simulink model "H2_DRI_plant"  (R2023b)
settings: Solver=ode15s  StartTime=0.0  StopTime=3600*24*5
values from neighbouring files (symbols this model uses):
  a_b = 6*(1-eps_bed)/(r_p*2)    (= 200)    [H2_DRI_plant_loader.m]
  A_furnace = pi*r_furnace^2    (= 23.7582944428)    [H2_DRI_plant_loader.m]
  A_furnace_pel = A_furnace*(1-eps_bed)    (= 11.8791472214)    [H2_DRI_plant_loader.m]
  A_wall = (2*pi*r_furnace*dz)    (= 1.1674837564)    [H2_DRI_plant_loader.m]
  c_CH4init = interp1([1:1:length(c_CH4init)],c_CH4init, linspace(1,length(c_CH4init),n_furnace))    [H2_DRI_plant_loader.m]    (also in inital_conditions.m = out.CH4_conc.data(end,:); initcond_H2.mat = [9.94099064213e-45 -4.26076213273e-25 -4.27813906239e-25 -4.; initcond_H2_PEM.mat = [4.30667282687e-45 4.29087427587e-45 3.8700760922e-45 3.7994)
  c_Cinit = interp1([1:1:length(c_Cinit)],c_Cinit, linspace(1,length(c_Cinit),n_furnace))    [H2_DRI_plant_loader.m]    (also in inital_conditions.m = out.C_conc.data(end,:); initcond_H2.mat = [1.45956980986e-305 6.99081092012e-307 8.03725154841e-309 -3; initcond_H2_PEM.mat = [1.92191536232e-321 1.91203404941e-321 1.97132192691e-321 1.)
  c_CO2init = interp1([1:1:length(c_CO2init)],c_CO2init, linspace(1,length(c_CO2init),n_furnace))    [H2_DRI_plant_loader.m]    (also in inital_conditions.m = out.CO2_conc.data(end,:); initcond_H2.mat = [1.40671287015e-53 9.99429922421e-25 1.00349747704e-24 1.007; initcond_H2_PEM.mat = [4.30579616214e-45 4.28998535938e-45 3.86916279543e-45 3.798)
  c_COinit = interp1([1:1:length(c_COinit)],c_COinit, linspace(1,length(c_COinit),n_furnace))    [H2_DRI_plant_loader.m]    (also in inital_conditions.m = out.CO_conc.data(end,:); initcond_H2.mat = [8.62168160047e-54 2.62488347241e-25 2.63562031881e-25 2.646; initcond_H2_PEM.mat = [-1.41770643933e-43 -1.41248114323e-43 -1.27321677334e-43 -1)
  c_Fe2O3init = interp1([1:1:length(c_Fe2O3init)],c_Fe2O3init, linspace(1,length(c_Fe2O3init),n_furnace))    [H2_DRI_plant_loader.m]    (also in inital_conditions.m = out.Fe2O3_conc.data(end,:); initcond_H2.mat = [-0.0576294325141 -0.0562977053664 -0.0549879883395 -0.05369; initcond_H2_PEM.mat = [-0.0421766495112 -0.0410731169681 -0.0399918101679 -0.03893)
  c_Fe3O4init = interp1([1:1:length(c_Fe3O4init)],c_Fe3O4init, linspace(1,length(c_Fe3O4init),n_furnace))    [H2_DRI_plant_loader.m]    (also in inital_conditions.m = out.Fe3O4_conc.data(end,:); initcond_H2.mat = [0.0460784397936 0.0452182842983 0.0443654100081 0.043519007; initcond_H2_PEM.mat = [0.0345314201173 0.0338401633931 0.0331554273597 0.032476466)
  c_Feinit = interp1([1:1:length(c_Feinit)],c_Feinit, linspace(1,length(c_Feinit),n_furnace))    [H2_DRI_plant_loader.m]    (also in inital_conditions.m = out.Fe_conc.data(end,:); initcond_H2.mat = [2291.15615825 2257.57098555 2219.35021937 2176.85237423 213; initcond_H2_PEM.mat = [2291.15370188 2257.40533074 2219.07663621 2176.56351656 213)
  c_FeOinit = interp1([1:1:length(c_FeOinit)],c_FeOinit, linspace(1,length(c_FeOinit),n_furnace))    [H2_DRI_plant_loader.m]    (also in inital_conditions.m = out.FeO_conc.data(end,:); initcond_H2.mat = [120.587032003 163.793602795 212.96382844 267.636483226 327.; initcond_H2_PEM.mat = [120.587036941 164.003608886 213.312732219 268.005087273 327)
  c_H2init = interp1([1:1:length(c_H2init)],c_H2init, linspace(1,length(c_H2init),n_furnace))    [H2_DRI_plant_loader.m]    (also in inital_conditions.m = out.H2_conc.data(end,:); initcond_H2.mat = [22.889073739 22.8842667021 22.8746324515 22.8599710419 22.8; initcond_H2_PEM.mat = [17.1469199078 17.1645959742 17.1787956185 17.1891948084 17.)
  c_H2Oinit = interp1([1:1:length(c_H2Oinit)],c_H2Oinit, linspace(1,length(c_H2Oinit),n_furnace))    [H2_DRI_plant_loader.m]    (also in inital_conditions.m = out.H2O_conc.data(end,:); initcond_H2.mat = [2.19324064628 2.2939246227 2.40633645516 2.52967076126 2.66; initcond_H2_PEM.mat = [0.652099757837 0.728496202531 0.813916572535 0.907739128718)
  c_N2init = interp1([1:1:length(c_N2init)],c_N2init, linspace(1,length(c_N2init),n_furnace))    [H2_DRI_plant_loader.m]    (also in inital_conditions.m = out.N2_conc.data(end,:); initcond_H2.mat = [0.439764167248 0.441445162144 0.443247144888 0.445152489232; initcond_H2_PEM.mat = [0.271051060899 0.272483637209 0.274000693264 0.275587826454)
  CCeaf = CC_eaf*TPDls*365    (= 195258297.6)    [H2_DRI_plant_loader.m]
  CCelect = CC_elect*MWelect*1000    (= 420000000)    [H2_DRI_plant_loader.m]
  CCsf = 49080*(TPDls*DRIsteel_conv/24*1000)^(0.6538)    (= 108365944.556)    [H2_DRI_plant_loader.m]
  CO2_diff_prop = [MM_CO2, 26.9]    [H2_DRI_plant_loader.m]
  CO_diff_prop = [MM_CO, 18.9]    [H2_DRI_plant_loader.m]
  dz = (h_furnace/(n_furnace-1))    (= 0.0675675675676)    [H2_DRI_plant_loader.m]
  eps_bed = 0.5    [H2_DRI_plant_loader.m]
  H2_diff_prop = [MM_H2, 2.31*2]    [H2_DRI_plant_loader.m]
  H2O_diff_prop = [MM_H2O, 13.1]    [H2_DRI_plant_loader.m]
  H2only = true    [H2_DRI_plant_loader.m]
  I_metal = P_metal/tau_metal    (= -0.00212856534696)    [H2_DRI_plant_loader.m]
  I_temp = P_metal/tau_temp    (= -0.00681140911026)    [H2_DRI_plant_loader.m]
  Kd = 5.29e-4    (= 0.000529)    [H2_DRI_plant_loader.m]
  Kmetal = -0.0435    [H2_DRI_plant_loader.m]
  MM_C = 12.011/1000    (= 0.012011)    [H2_DRI_plant_loader.m]
  MM_CH4 = 16.04    [H2_DRI_plant_loader.m]
  MM_CO = 28.01    [H2_DRI_plant_loader.m]
  MM_CO2 = 44.01    [H2_DRI_plant_loader.m]
  MM_Fe = 55.845/1000    (= 0.055845)    [H2_DRI_plant_loader.m]    (also in iron_props.m)
  MM_Fe2O3 = 159.69/1000    (= 0.15969)    [H2_DRI_plant_loader.m]    (also in iron_props.m)
  MM_Fe3O4 = 231.53/1000    (= 0.23153)    [H2_DRI_plant_loader.m]    (also in iron_props.m = 0.25153)
  MM_FeO = 71.844/1000    (= 0.071844)    [H2_DRI_plant_loader.m]    (also in iron_props.m)
  MM_H2 = 2.016    [H2_DRI_plant_loader.m]
  MM_H2O = 18.015    [H2_DRI_plant_loader.m]
  MM_N2 = 28.013    [H2_DRI_plant_loader.m]
  n_furnace = 75    [H2_DRI_plant_loader.m]
  ndotin = 2078.874    [H2_DRI_plant_loader.m]
  nr1init = interp1([1:1:length(nr1init)],nr1init, linspace(1,length(nr1init),n_furnace))    [H2_DRI_plant_loader.m]    (also in inital_conditions.m = out.nr1.data(end,:); initcond_H2.mat = [17138.9259823 17138.9192887 17138.9127057 17138.9062259 171; initcond_H2_PEM.mat = [17138.8483125 17138.8427658 17138.8373309 17138.8319998 171)
  nr2init = interp1([1:1:length(nr2init)],nr2init, linspace(1,length(nr2init),n_furnace))    [H2_DRI_plant_loader.m]    (also in inital_conditions.m = out.nr2.data(end,:); initcond_H2.mat = [11425.7909148 11425.7894343 11425.7880023 11425.7866166 114; initcond_H2_PEM.mat = [11425.7791649 11425.7778635 11425.776614 11425.7754137 1142)
  nr3init = interp1([1:1:length(nr3init)],nr3init, linspace(1,length(nr3init),n_furnace))    [H2_DRI_plant_loader.m]    (also in inital_conditions.m = out.nr3.data(end,:); initcond_H2.mat = [32930.1678524 32447.4572478 31898.1205118 31287.3104766 306; initcond_H2_PEM.mat = [32930.1325476 32445.0763361 31894.188375 31283.1588034 3061)
  P_gin = 101325*1.8    (= 182385)    [H2_DRI_plant_loader.m]
  P_metal = tau_metal/(Kmetal*tau_metal_desired)    (= -24.5210727969)    [H2_DRI_plant_loader.m]
  P_temp = tau_temp/(Kmetal*tau_temp_desired)    (= -45.9770114943)    [H2_DRI_plant_loader.m]
  R = 8.314    [Bou.m]    (also in H2_DRI_plant_loader.m; MD.m; SMR.m; USCM_CO.m)
  r_furnace = 2.75    [H2_DRI_plant_loader.m]
  r_p = 15e-3/2    (= 0.0075)    [H2_DRI_plant_loader.m]
  rho_p = 3528    [H2_DRI_plant_loader.m]
  Solids_In_Flow = 44.1    [H2_DRI_plant_loader.m]
  T_gin = 947 + 273    (= 1220)    [H2_DRI_plant_loader.m]
  T_ginit = interp1([1:1:length(T_ginit)],T_ginit, linspace(1,length(T_ginit),n_furnace))    [H2_DRI_plant_loader.m]    (also in inital_conditions.m = out.T_g.data(end,2:end); initcond_H2.mat = [1193.47241077 1188.60147936 1183.4413554 1178.04610025 1172; initcond_H2_PEM.mat = [1213.62674902 1206.86882145 1199.80656651 1192.51337179 118)
  T_sin = -10 + 273    (= 263)    [H2_DRI_plant_loader.m]
  T_sinit = interp1([1:1:length(T_sinit)],T_sinit, linspace(1,length(T_sinit),n_furnace))    [H2_DRI_plant_loader.m]    (also in inital_conditions.m = out.T_s.data(end,1:end-1); initcond_H2.mat = [1188.32225462 1183.11411515 1177.66723955 1172.0331792 1166; initcond_H2_PEM.mat = [1207.76768382 1200.67884676 1193.34151616 1185.82650883 117)
  tau = 1    [H2_DRI_plant_loader.m]
  tau_d = 3600*2    (= 7200)    [H2_DRI_plant_loader.m]
  tau_metal = 3.2*3600    (= 11520)    [H2_DRI_plant_loader.m]
  V_g = (4/3)*pi*r_p^3*n_pellets_dz*(eps_bed/(1-eps_bed))    (= 0.802645082526)    [H2_DRI_plant_loader.m]
  V_p = 4/3*pi*r_p^3    (= 1.76714586764e-06)    [H2_DRI_plant_loader.m]
  V_s = (4/3)*pi*r_p^3*n_pellets_dz    (= 0.802645082526)    [H2_DRI_plant_loader.m]
  w_Cin = 0    [H2_DRI_plant_loader.m]
  w_Fe2O3in = 0.9665    [H2_DRI_plant_loader.m]
  w_Fe3O4in = 0    [H2_DRI_plant_loader.m]
  w_Fein = 0    [H2_DRI_plant_loader.m]
  w_FeOin = 0    [H2_DRI_plant_loader.m]
  w_Ganin = 0.0335    [H2_DRI_plant_loader.m]
  x_CH4in = 0.105824828    [H2_DRI_plant_loader.m]
  x_CO2in = 0.024    [H2_DRI_plant_loader.m]
  x_COin = 0.320711862    [H2_DRI_plant_loader.m]
  x_H2in = 0.489526511    [H2_DRI_plant_loader.m]
  x_H2Oin = 0.042557156    [H2_DRI_plant_loader.m]
  x_N2in = 0.017379642    [H2_DRI_plant_loader.m]
libraries: slpidlib x3, simulink x1
(part 2 of 3)

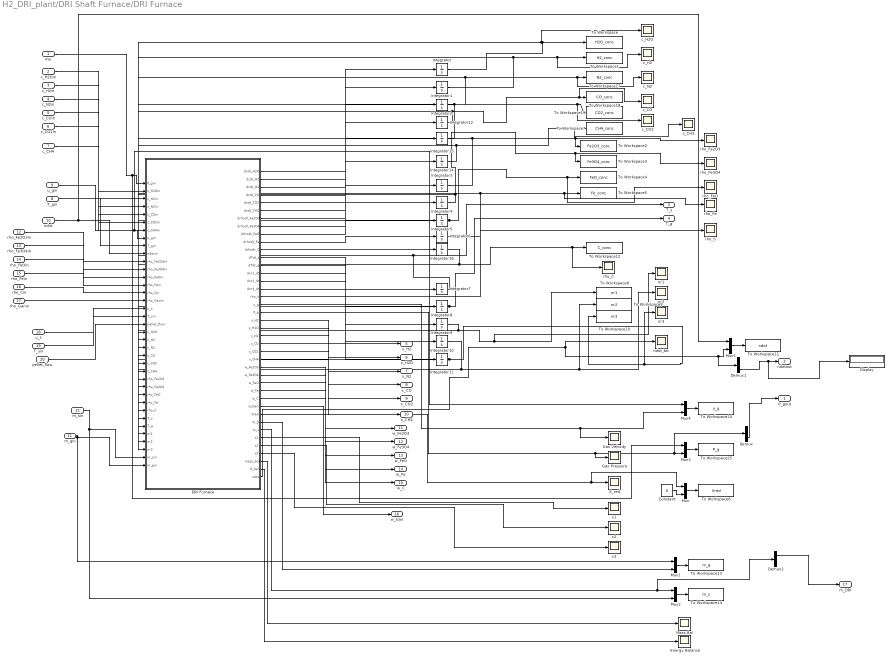
== system H2_DRI_plant/DRI Shaft Furnace/DRI Furnace ==
  Pin : Inport
  c_H2Oin : Inport  Port=2
  c_H2in : Inport  Port=3
  c_N2in : Inport  Port=4
  c_COin : Inport  Port=5
  c_CO2in : Inport  Port=6
  c_CH4 : Inport  Port=7
  T_gin : Inport  Port=8
  u_gin : Inport  Port=9
  ndot : Inport  Port=10
  m_gin : Inport  Port=11
  rho_Fe2O3in : Inport  Port=12
  rho_Fe3O4in : Inport  Port=13
  rho_FeOin : Inport  Port=14
  rho_Fein : Inport  Port=15
  rho_Cin : Inport  Port=16
  rho_Ganin : Inport  Port=17
  u_s : Inport  Port=18
  T_sin : Inport  Port=19
  pellet_flow : Inport  Port=20
  m_sin : Inport  Port=21
  Constant : Constant  Value=0
  DRI Furnace : MATLAB Function  TreatAsAtomicUnit=on
  Demux : Demux  Outputs=[n_furnace-1 1]
  Demux1 : Demux  Outputs=[n_furnace-1 1]
  Demux2 : Demux  Outputs=[1 n_furnace-1]
  Display : Display
  Energy Balance : Scope
  Gas Pressure : Scope
  Gas Velocity : Scope
  Integrator : Integrator  InitialCondition=c_H2Oinit
  Integrator1 : Integrator  InitialCondition=c_H2init
  Integrator10 : Integrator  InitialCondition=nr2init
  Integrator11 : Integrator  InitialCondition=nr3init
  Integrator12 : Integrator  InitialCondition=c_COinit
  Integrator13 : Integrator  InitialCondition=c_CO2init
  Integrator14 : Integrator  InitialCondition=c_CH4init
  Integrator16 : Integrator  InitialCondition=c_Cinit  AbsoluteTolerance=1e-4
  Integrator2 : Integrator  InitialCondition=c_N2init
  Integrator3 : Integrator  InitialCondition=c_Fe2O3init
  Integrator4 : Integrator  InitialCondition=c_Fe3O4init
  Integrator5 : Integrator  InitialCondition=c_FeOinit
  Integrator6 : Integrator  InitialCondition=c_Feinit
  Integrator7 : Integrator  InitialCondition=T_sinit
  Integrator8 : Integrator  InitialCondition=T_ginit
  Integrator9 : Integrator  InitialCondition=nr1init
  Mass Bal : Scope
  Mux{,1..5} (6 alike) : Mux  Inputs=2
  To Workspace : ToWorkspace  VariableName=H2O_conc  SaveFormat=Timeseries  SampleTime=-1
  To Workspace1 : ToWorkspace  VariableName=H2_conc  SaveFormat=Timeseries  SampleTime=-1
  To Workspace10 : ToWorkspace  VariableName=nr3  SaveFormat=Timeseries  SampleTime=-1
  To Workspace11 : ToWorkspace  VariableName=ndot  SaveFormat=Timeseries  SampleTime=-1
  To Workspace12 : ToWorkspace  VariableName=C_conc  SaveFormat=Timeseries  SampleTime=-1
  To Workspace13 : ToWorkspace  VariableName=m_g  SaveFormat=Timeseries  SampleTime=-1
  To Workspace14 : ToWorkspace  VariableName=m_s  SaveFormat=Timeseries  SampleTime=-1
  To Workspace17 : ToWorkspace  VariableName=N2_conc  SaveFormat=Timeseries  SampleTime=-1
  To Workspace18 : ToWorkspace  VariableName=CO_conc  SaveFormat=Timeseries  SampleTime=-1
  To Workspace19 : ToWorkspace  VariableName=CO2_conc  SaveFormat=Timeseries  SampleTime=-1
  To Workspace2 : ToWorkspace  VariableName=Fe2O3_conc  SaveFormat=Timeseries  SampleTime=-1
  To Workspace24 : ToWorkspace  VariableName=u_g  SaveFormat=Timeseries  SampleTime=-1
  To Workspace25 : ToWorkspace  VariableName=P_g  SaveFormat=Timeseries  SampleTime=-1
  To Workspace3 : ToWorkspace  VariableName=Fe3O4_conc  SaveFormat=Timeseries  SampleTime=-1
  To Workspace4 : ToWorkspace  VariableName=FeO_conc  SaveFormat=Timeseries  SampleTime=-1
  To Workspace5 : ToWorkspace  VariableName=Fe_conc  SaveFormat=Timeseries  SampleTime=-1
  To Workspace6 : ToWorkspace  VariableName=Xred  SaveFormat=Timeseries  SampleTime=-1
  To Workspace7 : ToWorkspace  VariableName=CH4_conc  SaveFormat=Timeseries  SampleTime=-1
  To Workspace8 : ToWorkspace  VariableName=nr1  SaveFormat=Timeseries  SampleTime=-1
  To Workspace9 : ToWorkspace  VariableName=nr2  SaveFormat=Timeseries  SampleTime=-1
  X_red : Scope
  c_CH3 : Scope
  c_CO : Scope
  c_CO2 : Scope
  c_H2 : Scope
  c_H2O : Scope
  c_N2 : Scope
  ndot_tot : Scope
  nr1 : Scope
  nr2 : Scope
  nr3 : Scope
  rho_C : Scope
  rho_Fe : Scope
  rho_Fe2O3 : Scope
  rho_Fe3O4 : Scope
  rho_FeO : Scope
  rho_S : Scope
  x1 : Scope
  x2 : Scope
  x3 : Scope
  P_gout : Outport
  ndotout : Outport  Port=2
  T_s : Outport  Port=3
  T_g : Outport  Port=4
  x_H2 : Outport  Port=5
  x_H2O : Outport  Port=6
  x_N2 : Outport  Port=7
  x_CO : Outport  Port=8
  x_CO2 : Outport  Port=9
  x_CH4 : Outport  Port=10
  w_Fe2O3 : Outport  Port=11
  w_Fe3O4 : Outport  Port=12
  w_FeO : Outport  Port=13
  w_Fe : Outport  Port=14
  w_C : Outport  Port=15
  w_Gan : Outport  Port=16
  m_DRI : Outport  Port=17
  wires:
  Integrator8/1 -> T_g/1, DRI Furnace/32(T_g)
  DRI Furnace/2(dcdt_H2) -> Integrator1/1
  Integrator10/1 -> To Workspace9/1, nr2/1, DRI Furnace/34(nr2)
  Integrator1/1 -> c_H2/1, To Workspace1/1, DRI Furnace/21(c_H2)
  m_sin/1 -> Mux2/2, DRI Furnace/36(m_sin)
  pellet_flow/1 -> DRI Furnace/19(pellet_flow)
  DRI Furnace/3(dcdt_N2) -> Integrator2/1
  Integrator9/1 -> To Workspace8/1, nr1/1, DRI Furnace/33(nr1)
  DRI Furnace/9(drhodt_FeO) -> Integrator5/1
  DRI Furnace/1(dcdt_H2O) -> Integrator/1
  rho_Fe2O3in/1 -> DRI Furnace/11(rho_Fe2O3in)
  DRI Furnace/10(drhodt_Fe) -> Integrator6/1
  Integrator7/1 -> T_s/1, DRI Furnace/31(T_s)
  Integrator4/1 -> rho_Fe3O4/1, To Workspace3/1, DRI Furnace/27(rho_Fe3O4)
  DRI Furnace/7(drhodt_Fe2O3) -> Integrator3/1
  Integrator3/1 -> DRI Furnace/26(rho_Fe2O3), rho_Fe2O3/1, To Workspace2/1
  DRI Furnace/13(dTdt_g) -> Integrator8/1
  DRI Furnace/15(dnr2_dt) -> Integrator10/1
  Integrator11/1 -> nr3/1, To Workspace10/1, DRI Furnace/35(nr3)
  DRI Furnace/16(dnr3_dt) -> Integrator11/1
  ndot/1 -> Mux5/1, DRI Furnace/10(ndotin)
  T_sin/1 -> DRI Furnace/18(T_sin)
  DRI Furnace/12(dTdt_s) -> Integrator7/1
  Integrator6/1 -> rho_Fe/1, To Workspace5/1, DRI Furnace/29(rho_Fe)
  rho_Fe3O4in/1 -> DRI Furnace/12(rho_Fe3O4in)
  DRI Furnace/38(mass_bal) -> Mass Bal/1
  T_gin/1 -> DRI Furnace/9(T_gin)
  Integrator2/1 -> c_N2/1, To Workspace17/1, DRI Furnace/22(c_N2)
  DRI Furnace/14(dnr1_dt) -> Integrator9/1
  rho_Fein/1 -> DRI Furnace/14(rho_Fein)
  Integrator/1 -> c_H2O/1, DRI Furnace/20(c_H2O), To Workspace/1
  u_s/1 -> DRI Furnace/17(u_s)
  DRI Furnace/8(drhodt_Fe3O4) -> Integrator4/1
  c_H2Oin/1 -> DRI Furnace/2(c_H2Oin)
  c_H2in/1 -> DRI Furnace/3(c_H2in)
  u_gin/1 -> DRI Furnace/8(u_gin), Mux4/1
  rho_FeOin/1 -> DRI Furnace/13(rho_FeOin)
  c_N2in/1 -> DRI Furnace/4(c_N2in)
  DRI Furnace/4(dcdt_CO) -> Integrator12/1
  DRI Furnace/5(dcdt_CO2) -> Integrator13/1
  Integrator13/1 -> c_CO2/1, To Workspace19/1, DRI Furnace/24(c_CO2)
  Integrator12/1 -> DRI Furnace/23(c_CO), c_CO/1, To Workspace18/1
  c_COin/1 -> DRI Furnace/5(c_COin)
  c_CO2in/1 -> DRI Furnace/6(c_CO2in)
  DRI Furnace/24(x_CO2) -> x_CO2/1
  DRI Furnace/23(x_CO) -> x_CO/1
  Integrator5/1 -> DRI Furnace/28(rho_FeO), rho_FeO/1, To Workspace4/1
  DRI Furnace/21(x_H2O) -> x_H2O/1
  DRI Furnace/20(x_H2) -> x_H2/1
  DRI Furnace/18(u_g) -> Gas Velocity/1, Mux4/2
  DRI Furnace/22(x_N2) -> x_N2/1
  DRI Furnace/26(w_Fe2O3) -> w_Fe2O3/1
  DRI Furnace/27(w_Fe3O4) -> w_Fe3O4/1
  DRI Furnace/28(w_FeO) -> w_FeO/1
  DRI Furnace/29(w_Fe) -> w_Fe/1
  DRI Furnace/19(P_g) -> Gas Pressure/1, Demux/1, Mux3/2
  DRI Furnace/34(m_s) -> Demux2/1, Mux2/1
  DRI Furnace/36(x2) -> x2/1
  DRI Furnace/37(x3) -> x3/1
  DRI Furnace/35(x1) -> x1/1
  c_CH4/1 -> DRI Furnace/7(c_CH4in)
  DRI Furnace/6(dcdt_CH4) -> Integrator14/1
  Integrator14/1 -> c_CH3/1, To Workspace7/1, DRI Furnace/25(c_CH4)
  DRI Furnace/25(x_CH4) -> x_CH4/1
  DRI Furnace/40(ndot) -> Demux1/1, Mux5/2, ndot_tot/1
  rho_Cin/1 -> DRI Furnace/15(rho_Cin)
  rho_Ganin/1 -> DRI Furnace/16(rho_Ganin)
  DRI Furnace/11(drhodt_C) -> Integrator16/1
  Integrator16/1 -> rho_C/1, To Workspace12/1, DRI Furnace/30(rho_C)
  DRI Furnace/30(w_C) -> w_C/1
  DRI Furnace/17(rho_s) -> rho_S/1
  DRI Furnace/31(w_Gan) -> w_Gan/1
  Constant/1 -> Mux/2
  Mux/1 -> To Workspace6/1
  Mux1/1 -> To Workspace13/1
  m_gin/1 -> Mux1/1, DRI Furnace/37(m_gin)
  DRI Furnace/33(m_g) -> Mux1/2
  Mux2/1 -> To Workspace14/1
  DRI Furnace/32(Xred) -> Mux/1, X_red/1
  DRI Furnace/39(Q_bal) -> Energy Balance/1
  Mux3/1 -> To Workspace25/1
  Mux4/1 -> To Workspace24/1
  Mux5/1 -> To Workspace11/1
  Pin/1 -> Mux3/1, DRI Furnace/1(P_gin)
  Demux/2 -> P_gout/1
  Demux1/2 -> Display/1, ndotout/1
  Demux2/1 -> m_DRI/1

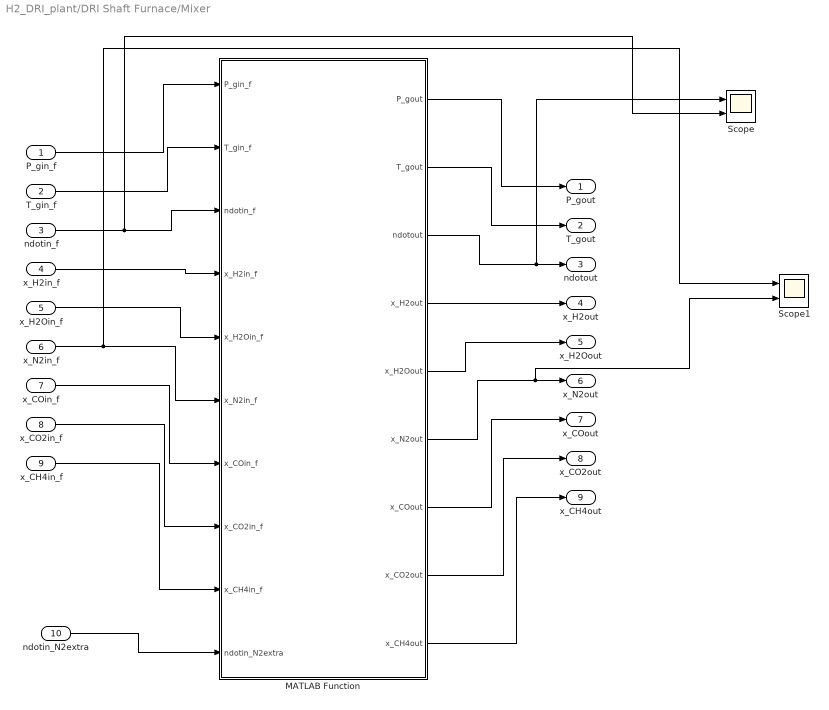
== system H2_DRI_plant/DRI Shaft Furnace/Mixer ==
  P_gin_f : Inport
  T_gin_f : Inport  Port=2
  ndotin_f : Inport  Port=3
  x_H2in_f : Inport  Port=4
  x_H2Oin_f : Inport  Port=5
  x_N2in_f : Inport  Port=6
  x_COin_f : Inport  Port=7
  x_CO2in_f : Inport  Port=8
  x_CH4in_f : Inport  Port=9
  ndotin_N2extra : Inport  Port=10
  MATLAB Function : MATLAB Function  TreatAsAtomicUnit=on
  Scope : Scope  NumInputPorts=2
  Scope1 : Scope  NumInputPorts=2
  P_gout : Outport
  T_gout : Outport  Port=2
  ndotout : Outport  Port=3
  x_H2out : Outport  Port=4
  x_H2Oout : Outport  Port=5
  x_N2out : Outport  Port=6
  x_COout : Outport  Port=7
  x_CO2out : Outport  Port=8
  x_CH4out : Outport  Port=9
  wires:
  MATLAB Function/1(P_gout) -> P_gout/1
  MATLAB Function/2(T_gout) -> T_gout/1
  MATLAB Function/3(ndotout) -> Scope/1, ndotout/1
  MATLAB Function/4(x_H2out) -> x_H2out/1
  MATLAB Function/5(x_H2Oout) -> x_H2Oout/1
  MATLAB Function/6(x_N2out) -> Scope1/2, x_N2out/1
  MATLAB Function/7(x_COout) -> x_COout/1
  MATLAB Function/8(x_CO2out) -> x_CO2out/1
  MATLAB Function/9(x_CH4out) -> x_CH4out/1
  ndotin_N2extra/1 -> MATLAB Function/10(ndotin_N2extra)
  x_CH4in_f/1 -> MATLAB Function/9(x_CH4in_f)
  x_CO2in_f/1 -> MATLAB Function/8(x_CO2in_f)
  x_COin_f/1 -> MATLAB Function/7(x_COin_f)
  x_N2in_f/1 -> Scope1/1, MATLAB Function/6(x_N2in_f)
  x_H2Oin_f/1 -> MATLAB Function/5(x_H2Oin_f)
  x_H2in_f/1 -> MATLAB Function/4(x_H2in_f)
  T_gin_f/1 -> MATLAB Function/2(T_gin_f)
  ndotin_f/1 -> Scope/2, MATLAB Function/3(ndotin_f)
  P_gin_f/1 -> MATLAB Function/1(P_gin_f)

== matlab function H2_DRI_plant/DRI Shaft Furnace/gas_conc ==
  data: P_gin input; c_H2Oin output; T_gin input; x_H2O input; x_H2 input; x_N2 input; x_CO input; x_CO2 input; x_CH4 input; A_furnace parameter; mol_flow input; c_H2in output; c_N2in output; c_COin output; c_CO2in output; c_CH4in output; R parameter; u_gin output; MM_H2O parameter; MM_N2 parameter; MM_H2 parameter; mol_flow output; eps_bed parameter; MM_CO parameter; MM_CO2 parameter; MM_CH4 parameter; m_gas output
function [c_H2Oin, c_H2in, c_N2in, c_COin, c_CO2in, c_CH4in, u_gin, mol_flow, m_gas] = gas_conc(P_gin, T_gin, x_H2O, x_H2, x_N2, x_CO, x_CO2, x_CH4, A_furnace, mol_flow, R, MM_H2O, MM_N2, MM_H2, eps_bed, MM_CO, MM_CO2, MM_CH4)

%toal molar concentration using ideal gas law
ct = P_gin/(R*T_gin); %mol/m^3 total

%molar concentrations of each gas species in
c_H2Oin = ct * x_H2O; %mol/m^3
c_H2in = ct * x_H2; %mol/m^3
c_N2in = ct * x_N2; %mol/m^3
c_COin = ct * x_CO; %mol/m^3
c_CO2in = ct * x_CO2; %mol/m^3
c_CH4in = ct * x_CH4; %mol/m^3


rho_H2Oin = c_H2Oin*MM_H2O/1000; %kg/m^3 total
rho_H2in = c_H2in*MM_H2/1000; %kg/m^3
rho_N2in = c_N2in*MM_N2/1000; %kg/m^3
rho_COin = c_COin*MM_CO/1000; %kg/m^3
rho_CO2in = c_CO2in*MM_CO2/1000; %kg/m^3
rho_CH4in = c_CH4in*MM_CO2/1000; %kg/m^3

w_totin = (c_H2in*MM_H2 + c_H2Oin*MM_H2O + c_N2in*MM_N2 + c_COin*MM_CO + c_CO2in*MM_CO2 + c_CH4in*MM_CH4);

w_H2in = c_H2in*MM_H2/w_totin;
w_H2Oin = c_H2Oin*MM_H2O /w_totin;
w_N2in = c_N2in*MM_N2/w_totin;
w_COin = c_COin*MM_CO/w_totin;
w_CO2in = c_CO2in*MM_CO2/w_totin;
w_CH4in = c_CH4in*MM_CH4/w_totin;



%mol_flow = m_gas*(w_H2Oin/(MM_H2O/1000) + w_H2in/(MM_H2/1000) + w_N2in/(MM_N2/1000) + w_COin/(MM_CO/1000) + w_CO2in/(MM_CO2/1000) + w_CH4in/(MM_CH4/1000)) ;
rho_gas = rho_H2Oin + rho_H2in + rho_N2in + rho_COin + rho_CO2in + rho_CH4in ; %kg/m^3 of GAS

m_gas = mol_flow*(x_H2*MM_H2 + x_CO*MM_CO + x_H2O*MM_H2O +x_CO2*MM_CO2 + x_N2*MM_N2 + x_CH4*MM_CH4)/1000; %kg/s

u_sup = m_gas/(rho_gas*A_furnace);

u_gin = u_sup/eps_bed;

== matlab function H2_DRI_plant/DRI Shaft Furnace/DRI Furnace/DRI Furnace ==
  data: P_gin input; c_H2Oin input; c_H2in input; c_N2in input; c_COin input; c_CO2in input; c_CH4in input; u_gin input; T_gin input; ndotin input; rho_Fe2O3in input; rho_Fe3O4in input; rho_FeOin input; rho_Fein input; rho_Cin input; rho_Ganin input; u_s input; T_sin input; pellet_flow input; c_H2O input; c_H2 input; c_N2 input; c_CO input; c_CO2 input; c_CH4 input; rho_Fe2O3 input; rho_Fe3O4 input; rho_FeO input; rho_Fe input; rho_C input; T_s input; T_g input; nr1 input; nr2 input; nr3 input; dcdt_H2O output; dcdt_H2 output; dcdt_N2 output; dcdt_CO output; dcdt_CO2 output; dcdt_CH4 output; drhodt_Fe2O3 output; drhodt_Fe3O4 output; drhodt_FeO output; drhodt_Fe output; drhodt_C output; dz parameter; n_furnace parameter; A_furnace parameter; r_p parameter; m_sin input; m_gin input; dTdt_s output; dTdt_g output; dnr1_dt output; dnr2_dt output; dnr3_dt output; a_b parameter; rho_s output; u_g output; P_g output; x_H2 output; x_H2O output; x_N2 output; x_CO output; x_CO2 output; x_CH4 output; w_Fe2O3 output; w_Fe3O4 output; w_FeO output; w_Fe output; w_C output; w_Gan output; Xred output; m_g output; m_s output; x1 output; x2 output; x3 output; mass_bal output; r_furnace parameter; A_wall parameter; A_furnace_pel parameter; eps_bed parameter; MM_H2O parameter; MM_H2 parameter; MM_N2 parameter; MM_Fe2O3 parameter; MM_Fe3O4 parameter; MM_FeO parameter; MM_Fe parameter; R parameter; V_g parameter; V_s parameter; MM_CO parameter; MM_CO2 parameter; Q_bal output; V_p parameter; MM_CH4 parameter; MM_C parameter; H2only parameter; CO2_diff_prop parameter; H2O_diff_prop parameter; H2_diff_prop parameter; CO_diff_prop parameter; ndot output
function [dcdt_H2O,dcdt_H2,dcdt_N2, dcdt_CO, dcdt_CO2, dcdt_CH4, drhodt_Fe2O3,drhodt_Fe3O4,drhodt_FeO,drhodt_Fe, drhodt_C, dTdt_s, dTdt_g, dnr1_dt,dnr2_dt,dnr3_dt, rho_s,...
    u_g, P_g, x_H2, x_H2O, x_N2, x_CO, x_CO2, x_CH4, w_Fe2O3, w_Fe3O4, w_FeO, w_Fe, w_C, w_Gan, Xred , m_g, m_s, x1, x2, x3, mass_bal, Q_bal, ndot]...
    = furnace(P_gin, c_H2Oin,c_H2in,c_N2in,c_COin, c_CO2in, c_CH4in, u_gin,T_gin, ndotin, rho_Fe2O3in,rho_Fe3O4in,rho_FeOin,rho_Fein, rho_Cin, rho_Ganin, u_s, T_sin, pellet_flow,...
    c_H2O,c_H2,c_N2,c_CO, c_CO2, c_CH4, rho_Fe2O3,rho_Fe3O4,rho_FeO,rho_Fe,rho_C, T_s, T_g, nr1, nr2, nr3, dz,n_furnace, A_furnace, r_p, m_sin,m_gin, a_b, r_furnace, A_wall,...
    A_furnace_pel, eps_bed, MM_H2O, MM_H2, MM_N2,MM_Fe2O3, MM_Fe3O4, MM_FeO, MM_Fe,R, V_g, V_s, MM_CO, MM_CO2, V_p, MM_CH4, MM_C, H2only, CO2_diff_prop, H2O_diff_prop, H2_diff_prop, CO_diff_prop)


% if iron oxide pellets contain more than Fe2O3 and gangue
% this will have to be changed or made as in inlet parameter
% moles of each species of iron oxide in
nr1in = 0;
nr2in = 0;
nr3in = 0;


% initialize a lot of different variables the size of the spatial nodes
w_H2 = zeros(size(rho_Fe2O3));
w_H2O = zeros(size(rho_Fe2O3));
w_N2 = zeros(size(rho_Fe2O3));
w_CO = zeros(size(rho_Fe2O3));
w_CO2 = zeros(size(rho_Fe2O3));
w_CH4 = zeros(size(rho_Fe2O3));

x_H2 = zeros(size(rho_Fe2O3));
x_H2O = zeros(size(rho_Fe2O3));
x_N2 = zeros(size(rho_Fe2O3));
x_CO = zeros(size(rho_Fe2O3));
x_CO2 = zeros(size(rho_Fe2O3));
x_CH4 = zeros(size(rho_Fe2O3));

mu_g = zeros(size(rho_Fe2O3));
Cp_g = zeros(size(rho_Fe2O3));
Pr_g = zeros(size(rho_Fe2O3));

rho_g = zeros(size(rho_Fe2O3));

Nu = zeros(size(rho_Fe2O3));
Re_p = zeros(size(rho_Fe2O3));

k_g = zeros(size(rho_Fe2O3));
h_sg = zeros(size(rho_Fe2O3));
U_wall = zeros(size(rho_Fe2O3));

D_H2_H2O = zeros(size(rho_Fe2O3));
D_CO_CO2 = zeros(size(rho_Fe2O3));

k_diff_H2 = zeros(size(rho_Fe2O3));
k_diff_CO = zeros(size(rho_Fe2O3));

rho_s = zeros(size(rho_Fe2O3));

w_Fe2O3 = zeros(size(rho_Fe2O3));
w_Fe3O4 = zeros(size(rho_Fe2O3));
w_FeO = zeros(size(rho_Fe2O3));
w_Fe = zeros(size(rho_Fe2O3));
w_C = zeros(size(rho_Fe2O3));
w_Gan = zeros(size(rho_Fe2O3));
Cp_s = zeros(size(rho_Fe2O3));

x1 = zeros(size(rho_Fe2O3));
x2 = zeros(size(rho_Fe3O4));
x3 = zeros(size(rho_FeO));
Xred = zeros(size(rho_FeO));

v1 = zeros(size(rho_Fe2O3));
v2 = zeros(size(rho_Fe3O4));
v3 = zeros(size(rho_FeO));
v4 = zeros(size(rho_Fe2O3));
v5 = zeros(size(rho_Fe3O4));
v6 = zeros(size(rho_FeO));
v7 = zeros(size(rho_FeO));
v8 = zeros(size(rho_FeO));
v9 = zeros(size(rho_FeO));
v10 = zeros(size(rho_FeO));

f1 = zeros(size(rho_Fe2O3));
f2 = zeros(size(rho_Fe3O4));
f3 = zeros(size(rho_FeO));

m_g = zeros(size(rho_Fe2O3));
m_s = zeros(size(rho_Fe2O3));

ct = zeros(size(rho_Fe2O3));

P_g = zeros(size(T_g));
ndot = zeros(size(c_H2O));


%initializing derivatives as zero to define size
dcdt_H2O = zeros(size(c_H2O));
dcdt_H2 = zeros(size(c_H2));
dcdt_N2 = zeros(size(c_N2));
dcdt_CO = zeros(size(c_CO));
dcdt_CO2 = zeros(size(c_CO2));
dcdt_CH4 = zeros(size(c_CH4));

drhodt_Fe2O3 = zeros(size(rho_Fe2O3));
drhodt_Fe3O4 = zeros(size(rho_Fe3O4));
drhodt_FeO = zeros(size(rho_FeO));
drhodt_Fe = zeros(size(rho_Fe));
drhodt_C = zeros(size(rho_Fe));

dnr1_dt = zeros(size(rho_Fe2O3));
dnr2_dt = zeros(size(rho_Fe3O4));
dnr3_dt = zeros(size(rho_FeO));
%dntot_dt = zeros(size(rho_FeO));

S_nr1 = zeros(size(rho_Fe2O3));
S_nr2 = zeros(size(rho_Fe3O4));
S_nr3 = zeros(size(rho_FeO));

u_g = zeros(size(rho_Fe2O3));

dTdt_s = zeros(size(T_s));
dTdt_g = zeros(size(T_g));

DelH1 = zeros(size(T_s));
DelH2 = zeros(size(T_s));
DelH3 = zeros(size(T_s));
DelH4 = zeros(size(T_s));
DelH5 = zeros(size(T_s));
DelH6 = zeros(size(T_s));
DelH7 = zeros(size(T_s));
DelH8 = zeros(size(T_s));


%% Inlet Gas and Iron Properties

% Weight fractions of each gas species
w_totin = (c_H2in*MM_H2 + c_H2Oin*MM_H2O + c_N2in*MM_N2 + c_COin*MM_CO + c_CO2in*MM_CO2 +  c_CH4in*MM_CH4);

w_H2in = c_H2in*MM_H2/w_totin;
w_H2Oin = c_H2Oin*MM_H2O /w_totin;
w_N2in = c_N2in*MM_N2/w_totin;
w_COin = c_COin*MM_CO/w_totin;
w_CO2in = c_CO2in*MM_CO2/w_totin;
w_CH4in = c_CH4in*MM_CH4/w_totin;

w_fracs = [w_H2in, w_H2Oin, w_N2in, w_COin, w_CO2in, w_CH4in]; % Create a vector of weight fractions for the prop_mix function

% Get properties from CoolProp interpolation based on temp of gas in
[rho_H2, mu_H2, k_H2, C_H2] = hydrogen(T_gin);
[rho_H2O, mu_H2O, k_H2O, C_H2O] = water(T_gin);
[rho_N2, mu_N2, k_N2, C_N2] = nitrogen(T_gin);
[rho_CO, mu_CO, k_CO, C_CO] = carbonmonoxide(T_gin);
[rho_CO2, mu_CO2, k_CO2, C_CO2] = carbondioxide(T_gin);
[rho_CH4, mu_CH4, k_CH4, C_CH4] = methane(T_gin);

% Create vectors of properties for prop_mix function
rhos = [rho_H2, rho_H2O, rho_N2, rho_CO, rho_CO2, rho_CH4];
mus = [mu_H2, mu_H2O, mu_N2, mu_CO, mu_CO2, mu_CH4];
ks = [k_H2, k_H2O, k_N2, k_CO, k_CO2, k_CH4];
Cps = [C_H2, C_H2O, C_N2, C_CO, C_CO2, C_CH4];

% get vicosicty and specific heat of gas mixture in
[~, mu_gin, ~,  Cp_gin] = prop_mix(rhos, mus, ks, Cps, w_fracs);

% density of gas coming from ideal gas law
rho_gin = ((c_H2in*MM_H2 + c_H2Oin*MM_H2O + c_N2in*MM_N2 + c_COin*MM_CO + c_CO2in*MM_CO2 + c_CH4in*MM_CH4 )/1000); %kg/m^3 of gas

% density of the iron pellets
rho_sin = rho_Fe2O3in + rho_Fe3O4in + rho_FeOin + rho_Fein + rho_Cin + rho_Ganin; %kg/m^3 of pellet in to the reactor

% weight fraction of each iron species at each spatial node
w_Fe2O3in =  rho_Fe2O3in/rho_sin;
w_Fe3O4in =  rho_Fe3O4in/rho_sin;
w_FeOin =  rho_FeOin/rho_sin;
w_Fein =  rho_Fein/rho_sin;
w_Cin =  rho_Cin/rho_sin;
w_Ganin =  rho_Ganin/rho_sin;

% specific heat of each iron species as a funciton of temperature of the solids
[Cps_iron, ~] = iron_props(T_sin); %J/kg-K, specific heat

% vector of weight fractions for mass weithed average
w_iron = [w_Fe2O3in, w_Fe3O4in, w_FeOin, w_Fein, w_Cin, w_Ganin];
Cp_sin = dot(Cps_iron, w_iron); %J/kg-K, mass weighted average of specific heat


%% Spatial Gas and Iron Properties 

for i = 1:n_furnace
    
    w_tot = (c_H2(i)*MM_H2 + c_H2O(i)*MM_H2O + c_N2(i)*MM_N2 + c_CO(i)*MM_CO + c_CO2(i)*MM_CO2 + c_CH4(i)*MM_CH4);

    % Weight fractions of each gas species for each spatial node
    w_H2(i) = c_H2(i)*MM_H2/w_tot;
    w_H2O(i) = c_H2O(i)*MM_H2O/w_tot; 
    w_N2(i) = c_N2(i)*MM_N2/w_tot; 
    w_CO(i) = c_CO(i)*MM_CO/w_tot;
    w_CO2(i) = c_CO2(i)*MM_CO2/w_tot;
    w_CH4(i) = c_CH4(i)*MM_CH4/w_tot;

    % density using molar concentrations
    rho_g(i) = ((c_H2(i)*MM_H2 + c_H2O(i)*MM_H2O + c_N2(i)*MM_N2 + c_CO(i)*MM_CO + c_CO2(i)*MM_CO2 + c_CH4(i)*MM_CH4)/1000); % kg/m^3 of gas, density of gas
    
    % mole fractions of each gas species for each spatial node
    ct(i) = c_H2(i) + c_H2O(i) + c_N2(i) + c_CO(i) + c_CO2(i) + c_CH4(i);
    x_H2(i) = c_H2(i)/ct(i);
    x_H2O(i) = c_H2O(i)/ct(i);
    x_N2(i) = c_N2(i)/ct(i);
    x_CO(i) = c_CO(i)/ct(i);
    x_CO2(i) = c_CO2(i)/ct(i);
    x_CH4(i) = c_CH4(i)/ct(i);
    
    % Create vectors of weight frac for prop_mix function
    w_fracs = [w_H2(i), w_H2O(i), w_N2(i), w_CO(i), w_CO2(i), w_CH4(i)];

    % Get properties from CoolProp interpolation based on temp of gas at each spatial node
    [rho_H2, mu_H2, k_H2, C_H2] = hydrogen(T_g(i));
    [rho_H2O, mu_H2O, k_H2O, C_H2O] = water(T_g(i));
    [rho_N2, mu_N2, k_N2, C_N2] = nitrogen(T_g(i));
    [rho_CO, mu_CO, k_CO, C_CO] = carbonmonoxide(T_gin);
    [rho_CO2, mu_CO2, k_CO2, C_CO2] = carbondioxide(T_gin);
    [rho_CH4, mu_CH4, k_CH4, C_CH4] = methane(T_gin);
    
    % Create vectors of properties for prop_mix function
    rhos = [rho_H2, rho_H2O, rho_N2, rho_CO, rho_CO2, rho_CH4];
    mus = [mu_H2, mu_H2O, mu_N2, mu_CO, mu_CO2, mu_CH4];
    ks = [k_H2, k_H2O, k_N2, k_CO, k_CO2, k_CH4];
    Cps = [C_H2, C_H2O, C_N2, C_CO, C_CO2, C_CH4];

    % get vicosicty, thermal conductivity, specific heat of gas mixture at each spatial node
    [~, mu_g(i), k_g(i), Cp_g(i)] = prop_mix(rhos, mus, ks, Cps, w_fracs);
    
    % density of the iron pellets
    rho_s(i) = rho_Fe2O3(i) + rho_Fe3O4(i) + rho_FeO(i) + rho_Fe(i) + rho_C(i) + rho_Ganin; %kg/m^3 of pellet
    
    % weight fraction of each iron species at each spatial node
    w_Fe2O3(i) =  rho_Fe2O3(i)/rho_s(i);
    w_Fe3O4(i) =  rho_Fe3O4(i)/rho_s(i);
    w_FeO(i) =  rho_FeO(i)/rho_s(i);
    w_Fe(i) =  rho_Fe(i)/rho_s(i);
    w_C(i) =  rho_C(i)/rho_s(i);
    w_Gan(i) =  rho_Ganin/rho_s(i);

    % specific heat of each iron species as a funciton of temperature of the solids
    [Cps_iron, ~] = iron_props(T_s(i)); %J/kg-K, specific heat
    
    % vector of weight fractions for mass weithed average
    w_iron = [w_Fe2O3(i), w_Fe3O4(i), w_FeO(i), w_Fe(i), w_C(i), w_Gan(i)];
    Cp_s(i) = dot(Cps_iron, w_iron); %J/kg-K, mass weighted average of specific heat

end



%% Rate of Reaction using Unreacted Shrinking Core Model

% C ratio from Chipman's relationship
Cratio = (w_C./(MM_C))./(w_Fe./MM_Fe);
Cratio(Cratio<1e-5) = 1e-5;

% find moles of each iron species available for reaction
mol_Fe2O3 = rho_Fe2O3in/MM_Fe2O3*V_s;
mol_Fe3O4 = mol_Fe2O3*(2/3); % 2/3 from stoichiometry 
mol_FeO = mol_Fe3O4*(3/1); % 3/1 from stoichiometry


%if H2only == false

for i = 1:n_furnace

    % f values are fraction of moles that have reacted for each nr which is moles reacted down the length of the reactor
    f1(i) = nr1(i)/mol_Fe2O3;
    f2(i) = nr2(i)/mol_Fe3O4;
    f3(i) = nr3(i)/mol_FeO;
    
    % fraction of moles available to react
    a = 1-f1(i);
    b = 1-f2(i);
    c = 1-f3(i);
    
    % make sure we aren't slighlty negative from rounding etc. as this will cause errors
    a(a<1e-10) = 1e-10;
    b(b<1e-10) = 1e-10;
    c(c<1e-10) = 1e-10;
    
    % x values are used in the unreacted shrinking core model (USCM)
    % x values are the radius of unreacted iron species for each reaction
    % divided by radius of the pellet
    % x values of zero mean that that iron reaction has fully reacted
    % the 1/3 comes from geometry of a sphere
    x1(i) = (a).^(1/3); % radius of Fe3O4/Fe2O3
    x2(i) = (b).^(1/3); % radius of FeO/Fe3O4
    x3(i) = (c).^(1/3); % radisu of Fe/FeO
    
    % Fractional reduction of iron oxide (F in paper)
    % 1 = all iron oxide species have been reduced
    Xred(i) = 1 -((1/9)*x1(i) + (2/9)*x1(i) + (6/9)*x3(i)); 

    % these are the other gases (ogs) to account for in equilbrium values
    % for the USCM
    x_H2_ogs = 1 - x_CO(i) - x_CO2(i) - x_N2(i) - x_CH4(i);
    x_CO_ogs = 1 - x_H2(i) - x_H2O(i) - x_N2(i) - x_CH4(i);  

    if i == 1
        u_gin = (ndotin*R*T_gin)/(P_gin*eps_bed*A_furnace); % m/s, interstitial gas flow in

        % average properties for Ergun eq.
        mu_gavg = (mu_gin + mu_g(i))/2;
        rho_gavg = (rho_gin + rho_g(i))/2;
        
        %P drop using Ergun equation and velocicty at node upwind
        P_g(i) = -((150*(1-eps_bed)^2*mu_gavg*u_gin)/((2*r_p)^2*eps_bed^2)+(1.75*rho_gavg*(1-eps_bed)*u_gin^2)/(2*r_p*eps_bed))*dz + P_gin; % Pa, pressure of gas at node 1
           
        D_H2_H2O(i) = fuller(H2O_diff_prop, H2_diff_prop, T_g(i), P_g(i)); % m^2/s, diffusion coefficent of H2O/H2 at gas temp and pressure for each spatial node
        D_CO_CO2(i) = fuller(CO_diff_prop, CO2_diff_prop, T_g(i), P_g(i)); % m^2/s, diffusion coefficent of H2O/H2 at gas temp and pressure for each spatial node
        
        mu_kine = mu_g(i)/rho_g(i); %m^2/2, kinematic viscosity of gas
        
        Sc = mu_kine/D_H2_H2O(i); % unitless, Schmidt number
        Sh = 2 + 0.39*Re_p(i)^(1/2)*Sc^(1/3); % unitless, Sherwood number of diffusion of gas to pellet film
        
        k_diff_H2(i) = Sh*D_H2_H2O(i)/(2*r_p); % m/s, mass tranfer coefficient of gas to pellet
        k_diff_CO(i) = Sh*D_CO_CO2(i)/(2*r_p); % m/s, mass tranfer coefficient of gas to pellet

        %Rate of reaction for three seperate reactions 1, 2, 3 using unreacted
        %shrinking core model in mol H2 per s per pellet
        [v1(i), v2(i), v3(i)] = USCM_H2(x1(i),x2(i),x3(i), r_p, T_s(i), c_H2(i), ct(i), x_H2_ogs, k_diff_H2(i)); %mol H2 per s per pellet
        
        if H2only == false % if H2only = false then include all rxns with carbon
            [v4(i), v5(i), v6(i)] = USCM_CO(x1(i),x2(i),x3(i), r_p, T_s(i), c_CO(i), ct(i), x_CO_ogs, k_diff_CO(i)); %mol CO per s per pellet
            v7(i) = WGS(Xred(i), T_g(i), P_g(i), V_p, x_H2(i), x_H2O(i), x_CO(i), x_CO2(i)); %mol CO/H2O per s per pellet
            v8(i) = SMR(Xred(i), T_g(i), P_g(i), V_p, x_H2(i), x_H2O(i), x_CO(i), x_CH4(i));  %mol CH4/H2O per s per pellet  
            v9(i) = MD(Xred(i), T_s(i), P_g(i), V_p, x_H2(i), x_CH4(i), Cratio(i)); %mol CH4 per s per pellet
            v10(i) = Bou(Xred(i), T_s(i), P_g(i), V_p, x_H2(i), x_CO(i), x_CO2(i), Cratio(i)); %mol CO per s per pellet
        
        else %otherwise only reactions are H2 iron oxide rxns from USCM
            v4(i) = 0;
            v5(i) = 0;
            v6(i) = 0;
            v7(i) = 0;
            v8(i) = 0;
            v9(i) = 0;
            v10(i) = 0;
        end

        ndot(i) = ndotin + (2*v8(i) + v9(i) - v10(i))*(pellet_flow*dz/u_s); %mol/s

        % velocity using ideal gas law coupled with Ergun eq. 
        u_g(i) = (ndot(i)*R*T_g(i))/(P_g(i)*eps_bed*A_furnace); % m/s, interstitial gas flow in

    else

        % average properties for Ergun eq.
        mu_gavg = (mu_g(i-1) + mu_g(i))/2;
        rho_gavg = (rho_g(i-1) + rho_g(i))/2;

        %P drop using Ergun equation and velocicty at node upwind
        P_g(i) = -((150*(1-eps_bed)^2*mu_gavg*u_g(i-1))/((2*r_p)^2*eps_bed^2)+(1.75*rho_gavg*(1-eps_bed)*u_g(i-1)^2)/(2*r_p*eps_bed))*dz + P_g(i-1);
        P_g(P_g<0.1*101325) = 0.1*101325; %just helps fix errors at begining of sims.
        
        D_H2_H2O(i) = fuller(H2O_diff_prop, H2_diff_prop, T_g(i), P_g(i)); % m^2/s, diffusion coefficent of H2O/H2 at gas temp and pressure for each spatial node
        D_CO_CO2(i) = fuller(CO_diff_prop, CO2_diff_prop, T_g(i), P_g(i)); % m^2/s, diffusion coefficent of H2O/H2 at gas temp and pressure for each spatial node
        
        mu_kine = mu_g(i)/rho_g(i); %m^2/2, kinematic viscosity of gas
        
        Sc = mu_kine/D_H2_H2O(i); % unitless, Schmidt number
        Sh = 2 + 0.39*Re_p(i)^(1/2)*Sc^(1/3); % unitless, Sherwood number of diffusion of gas to pellet film
        
        k_diff_H2(i) = Sh*D_H2_H2O(i)/(2*r_p); % m/s, mass tranfer coefficient of gas to pellet
        k_diff_CO(i) = Sh*D_CO_CO2(i)/(2*r_p); % m/s, mass tranfer coefficient of gas to pellet

        %Rate of reaction for three seperate reactions 1, 2, 3 using unreacted
        %shrinking core model in mol H2 per s per pellet
        [v1(i), v2(i), v3(i)] = USCM_H2(x1(i),x2(i),x3(i), r_p, T_s(i), c_H2(i), ct(i), x_H2_ogs, k_diff_H2(i)); %mol H2 per s per pellet
        
        if H2only == false % if H2only = false then include all rxns with carbon
            [v4(i), v5(i), v6(i)] = USCM_CO(x1(i),x2(i),x3(i), r_p, T_s(i), c_CO(i), ct(i), x_CO_ogs, k_diff_CO(i)); %mol CO per s per pellet
            v7(i) = WGS(Xred(i), T_g(i), P_g(i), V_p, x_H2(i), x_H2O(i), x_CO(i), x_CO2(i)); %mol CO/H2O per s per pellet
            v8(i) = SMR(Xred(i), T_g(i), P_g(i), V_p, x_H2(i), x_H2O(i), x_CO(i), x_CH4(i));  %mol CH4/H2O per s per pellet  
            v9(i) = MD(Xred(i), T_s(i), P_g(i), V_p, x_H2(i), x_CH4(i), Cratio(i)); %mol CH4 per s per pellet
            v10(i) = Bou(Xred(i), T_s(i), P_g(i), V_p, x_H2(i), x_CO(i), x_CO2(i), Cratio(i)); %mol CO per s per pellet
        
        else %otherwise only reactions are H2 iron oxide rxns from USCM
            v4(i) = 0;
            v5(i) = 0;
            v6(i) = 0;
            v7(i) = 0;
            v8(i) = 0;
            v9(i) = 0;
            v10(i) = 0;
        end

        ndot(i) = ndot(i-1) + (2*v8(i) + v9(i) - v10(i))*(pellet_flow*dz/u_s); %mol/s

        % velocity using ideal gas law coupled with Ergun eq. 
        u_g(i) = (ndot(i)*R*T_g(i))/(P_g(i)*eps_bed*A_furnace); % m/s, interstitial gas flow in
        
    end
end

% sometimes will get small negative values for the USCM
% it is modeled as only a heterogenous forward rxn
v1(v1<0) = 0;
v2(v2<0) = 0;
v3(v3<0) = 0;
v4(v4<0) = 0;
v5(v5<0) = 0;
v6(v6<0) = 0;

%% Source Terms from Reaction

% Source terms of each gas from reactions -- mol/m^3 gas*s
S_H2O = (v1 + v2 + v3 - v7 - v8)*(pellet_flow/(A_furnace_pel*u_s))*((1-eps_bed)/eps_bed); %mol/m^3 gas *s
S_H2 = (-v1 - v2 - v3 + v7 + 3*v8 + 2*v9)*(pellet_flow/(A_furnace_pel*u_s))*((1-eps_bed)/eps_bed); %mol/m^3 gas *s
S_CO2 = (v4 + v5 + v6 + v7 + v10)*(pellet_flow/(A_furnace_pel*u_s))*((1-eps_bed)/eps_bed); %mol/m^3 gas *s
S_CO = (-v4 - v5 - v6 - v7 + v8 - 2*v10)*(pellet_flow/(A_furnace_pel*u_s))*((1-eps_bed)/eps_bed); %mol/m^3 gas *s
S_CH4 = (-v8 - v9)*(pellet_flow/(A_furnace_pel*u_s))*((1-eps_bed)/eps_bed); %mol/m^3 gas *s

% Source terms of each iron species : note that molar masses are in kg/mol 
S_Fe2O3 = -3*MM_Fe2O3*(v1+v4) * (pellet_flow/(A_furnace_pel*u_s)); % kg/m^3 solid*s
S_Fe3O4 = MM_Fe3O4*(2*(v1+v4) - (v2+v5)) * (pellet_flow/(A_furnace_pel*u_s));  % kg/m^3 solid*s
S_FeO = MM_FeO*(3*(v2+v5) - (v3+v6))* (pellet_flow/(A_furnace_pel*u_s));  % kg/m^3 solid*s
S_Fe = MM_Fe*(v3+v6) * (pellet_flow/(A_furnace_pel*u_s)); % kg/m^3 solid*s
S_C = MM_C*(v9 + v10)*(pellet_flow/(A_furnace_pel*u_s)); %kg/m^3 solid *s

% Source terms of each moles of iron species reacted!
% Used to track a dynamic X values
for i = 1:n_furnace
    S_nr1(i) = 3*(v1(i)+v4(i))*(pellet_flow*dz/u_s); % moles/s Fe2O3 reacted
    S_nr2(i) = (v2(i)+v5(i))*(pellet_flow*dz/u_s);  % moles/s Fe3O4 reacted
    S_nr3(i) = (v3(i)+v6(i))*(pellet_flow*dz/u_s); % moles/s FeO reacted
end


%% Heat Transfer Coefficients

for i = 1:n_furnace
    Pr_g(i) = Cp_g(i)*mu_g(i)/k_g(i); % unitless, Prandlt number of gas

    Re_p(i) = (rho_g(i)*u_g(i)*2*r_p)/mu_g(i); % unitless, Reynolds number of gas using pellet diameter as characteristic length
    
    Nu(i) = 2 + 0.39*Re_p(i)^(1/2)*Pr_g(i)^(1/3); % unitless, Nusselt number of heat transfer from gas to solid
    h_sg(i) = Nu(i)*k_g(i)/(2*r_p); % W/m^2-K, convective heat transfer coeffient of solid to gas
 
    U_wall(i) = (2.26 * Re_p(i)^0.8*Pr_g(i)^(1/3)*exp((-12*r_p)/(2*r_furnace)))*((mu_g(i)/rho_g(i))/(2*r_furnace));% W/m^2-K, convective heat transfer coeffient of gas to wall

end


%% Mass Balances
%Accounts for advective transport and reaction

for i = 1:n_furnace
    
    if  i == 1
        
        % change in concentrtation of each gas species, mol/m^3-s
        dcdt_H2O(i) = (u_gin*c_H2Oin - u_g(i)*c_H2O(i))/dz + S_H2O(i);
        dcdt_H2(i) = (u_gin*c_H2in - u_g(i)*c_H2(i))/dz + S_H2(i);
        dcdt_N2(i) = (u_gin*c_N2in - u_g(i)*c_N2(i))/dz;
        dcdt_CO(i) = (u_gin*c_COin - u_g(i)*c_CO(i))/dz + S_CO(i);
        dcdt_CO2(i) = (u_gin*c_CO2in - u_g(i)*c_CO2(i))/dz + S_CO2(i);
        dcdt_CH4(i) = (u_gin*c_CH4in - u_g(i)*c_CH4(i))/dz + S_CH4(i);

        m_g(i) = rho_g(i)*V_g*u_g(i)/dz; % kg/s, mass flow rate of gas

    else
     
        % change in concentrtation of each gas species, mol/m^3-s
        dcdt_H2O(i) = (u_g(i-1)*c_H2O(i-1) - u_g(i)*c_H2O(i))/dz + S_H2O(i);
        dcdt_H2(i) = (u_g(i-1)*c_H2(i-1) - u_g(i)*c_H2(i))/dz + S_H2(i);
        dcdt_N2(i) = (u_g(i-1)*c_N2(i-1) - u_g(i)*c_N2(i))/dz;
        dcdt_CO(i) = (u_g(i-1)*c_CO(i-1) - u_g(i)*c_CO(i))/dz + S_CO(i);
        dcdt_CO2(i) = (u_g(i-1)*c_CO2(i-1) - u_g(i)*c_CO2(i))/dz + S_CO2(i);
        dcdt_CH4(i) = (u_g(i-1)*c_CH4(i-1) - u_g(i)*c_CH4(i))/dz + S_CH4(i);

        m_g(i) = rho_g(i)*V_g*u_g(i)/dz; % kg/s, mass flow rate of gas

    end

end

for i = 1:n_furnace

    if i == n_furnace

        % change in solid mass concentration in kg/m^3-s
        %Fe2O3
        drhodt_Fe2O3(i) = (u_s/dz)*(rho_Fe2O3in - rho_Fe2O3(i)) + S_Fe2O3(i);
        %Fe3O4
        drhodt_Fe3O4(i) = (u_s/dz)*(rho_Fe3O4in - rho_Fe3O4(i)) + S_Fe3O4(i);
        %FeO
        drhodt_FeO(i) = (u_s/dz)*(rho_FeOin - rho_FeO(i)) + S_FeO(i);
        %Fe
        drhodt_Fe(i) = (u_s/dz)*(rho_Fein - rho_Fe(i)) + S_Fe(i); 
        %C
        drhodt_C(i) = (u_s/dz)*(rho_Cin - rho_C(i)) + S_C(i); 
                
        m_s(i) = rho_s(i)*V_s*u_s/dz; % kg/s, mass flow rate of solid

    else

        % change in solid mass concentration in kg/m^3-s
        %Fe2O3
        drhodt_Fe2O3(i) = (u_s/dz)*(rho_Fe2O3(i+1) - rho_Fe2O3(i)) + S_Fe2O3(i);
        %Fe3O4
        drhodt_Fe3O4(i) = (u_s/dz)*(rho_Fe3O4(i+1) - rho_Fe3O4(i)) + S_Fe3O4(i);
        %FeO
        drhodt_FeO(i) = (u_s/dz)*(rho_FeO(i+1) - rho_FeO(i)) + S_FeO(i);
        %Fe
        drhodt_Fe(i) = (u_s/dz)*(rho_Fe(i+1) - rho_Fe(i)) + S_Fe(i);
        %C
        drhodt_C(i) = (u_s/dz)*(rho_C(i+1) - rho_C(i)) + S_C(i); 
       
        m_s(i) = rho_s(i)*V_s*u_s/dz; % kg/s, mass flow rate of solid

    end

end

% moles of each iron oxide reacted per second
% used in X calculation
for i = 1:n_furnace

    if i == n_furnace
        % mole/s reacted from each iron reaction
        %nr1
        dnr1_dt(i) = (u_s/dz)*(nr1in - nr1(i)) + S_nr1(i);
        %nr2
        dnr2_dt(i) = (u_s/dz)*(nr2in - nr2(i)) + S_nr2(i);
        %nr3
        dnr3_dt(i) = (u_s/dz)*(nr3in - nr3(i)) + S_nr3(i);

    else
        
        % mole/s reacted from each iron reaction
        %nr1
        dnr1_dt(i) = (u_s/dz)*(nr1(i+1) - nr1(i)) + S_nr1(i);
        %nr2
        dnr2_dt(i) = (u_s/dz)*(nr2(i+1) - nr2(i)) + S_nr2(i);
        %nr3
        dnr3_dt(i) = (u_s/dz)*(nr3(i+1) - nr3(i)) + S_nr3(i);

    end
end


% Mass balance checks all in kg/s
m_sout = m_s(1);
m_gout = m_g(n_furnace);

mass_in = m_gin + m_sin;
mass_out = m_gout + m_sout;

mass_bal = mass_in - mass_out;

%% Energy Balance

T_amb = 25+273; %K, constant for now, but can be made in input, has small effect due to fast gas residence time

for i = 1:n_furnace
    
    % heats of reaction for each reaction

    % endothermic overall Deh1 is exothermic - from A. Rahimi, A. Niksiar / International Journal of Mineral Processing 124 (2013) 58–66
    % J/mol H2
    DelH1(i) = 18437.9 -102.28*T_s(i) + 0.097044*T_s(i)^2;
    DelH2(i) = 52360.5 +73.29*T_s(i) - 0.096454*T_s(i)^2; 
    DelH3(i) = 40087.4 -44.66*T_s(i) + 0.023847*T_s(i)^2;
    
    % J/mol CO
    % all exothermic - from A. Rahimi, A. Niksiar / International Journal of Mineral Processing 124 (2013) 58–66
    DelH4(i) = -26177.6 -92.125*T_s(i) + 0.096808*T_s(i)^2;
    DelH5(i)  = 7744.5 +83.5404*T_s(i) - 0.09669*T_s(i)^2;
    DelH6(i) = -4527.4 -34.5157*T_s(i) + 0.023612*T_s(i)^2;
    
    % J/mol CO/H2O
    DelH7(i) = (-10000 + 2.31*(T_g(i) -273))*4.184; %exothermic, from Takahashi, R., Takahashi, Y., Yagi, J., & Omori, Y. (1986). Operation and Simulation of Pressurized Shaft Furnace for Direct Reduction. Transactions of the Iron and Steel Institute of Japan, 26(9), 765–774.
    % J/mol CH4/H2O
    DelH8(i) = (-0.0227*T_g(i)^2 + 54.845*T_g(i) + 193245); % endothermic, CoolProp regression
    
    DelH9 = 75.4e3; % J/mol CH4 endothermic
    DelH10 = -172000; %J/mol CO, exothermic

    if i == 1
        % K/s, temp change of solid and gas
        dTdt_s(i) = (m_s(i+1)*Cp_s(i+1))/(rho_s(i)*Cp_s(i)*V_s)*T_s(i+1) - m_s(i)/(rho_s(i)*V_s)*T_s(i)...   
        - ((h_sg(i)*3)/(rho_s(i)*Cp_s(i)*r_p))*(T_s(i)-T_g(i)) + ...
          (1/(rho_s(i)*Cp_s(i)))*(-v1(i)*DelH1(i) -v2(i)*DelH2(i) -v3(i)*DelH3(i) - v4(i)*DelH4(i) -v5(i)*DelH5(i) -v6(i)*DelH6(i) -v9(i)*DelH9 - v10(i)*DelH10)*(pellet_flow/(A_furnace_pel*u_s));
      
   
       dTdt_g(i) = (m_gin*Cp_gin)/(rho_g(i)*Cp_g(i)*V_g)*T_gin - m_g(i)/(rho_g(i)*V_g)*T_g(i)...   
        - ((h_sg(i)*a_b)/(rho_g(i)*Cp_g(i)*eps_bed))*(T_g(i)-T_s(i))...
        - ((U_wall(i)*A_wall)/(rho_g(i)*Cp_g(i)*V_g))*(T_g(i)-T_amb)...
        + (1/(rho_g(i)*Cp_g(i)))*(-v7(i)*DelH7(i) - v8(i)*DelH8(i))*(pellet_flow/(A_furnace_pel*u_s));



    elseif i == n_furnace
        
        % K/s, temp change of solid and gas
        dTdt_s(i) = (m_sin*Cp_sin)/(rho_s(i)*Cp_s(i)*V_s)*T_sin - m_s(i)/(rho_s(i)*V_s)*T_s(i)...   
        - ((h_sg(i)*3)/(rho_s(i)*Cp_s(i)*r_p))*(T_s(i)-T_g(i)) + ... 
          (1/(rho_s(i)*Cp_s(i)))*(-v1(i)*DelH1(i) -v2(i)*DelH2(i) -v3(i)*DelH3(i) - v4(i)*DelH4(i) -v5(i)*DelH5(i) -v6(i)*DelH6(i) -v9(i)*DelH9 - v10(i)*DelH10)*(pellet_flow/(A_furnace_pel*u_s));
       

        dTdt_g(i) = (m_g(i-1)*Cp_g(i-1))/(rho_g(i)*Cp_g(i)*V_g)*T_g(i-1) - m_g(i)/(rho_g(i)*V_g)*T_g(i)...   
          - ((h_sg(i)*a_b)/(rho_g(i)*Cp_g(i)*eps_bed))*(T_g(i)-T_s(i))...
          - ((U_wall(i)*A_wall)/(rho_g(i)*Cp_g(i)*V_g))*(T_g(i)-T_amb)...
          + (1/(rho_g(i)*Cp_g(i)))*(-v7(i)*DelH7(i) - v8(i)*DelH8(i))*(pellet_flow/(A_furnace_pel*u_s));


    else
        
        % K/s, temp change of solid and gas
        dTdt_s(i) = (m_s(i+1)*Cp_s(i+1))/(rho_s(i)*Cp_s(i)*V_s)*T_s(i+1) - m_s(i)/(rho_s(i)*V_s)*T_s(i)...   
        - ((h_sg(i)*3)/(rho_s(i)*Cp_s(i)*r_p))*(T_s(i)-T_g(i))+ ...
          (1/(rho_s(i)*Cp_s(i)))*(-v1(i)*DelH1(i) -v2(i)*DelH2(i) -v3(i)*DelH3(i) - v4(i)*DelH4(i) -v5(i)*DelH5(i) -v6(i)*DelH6(i) -v9(i)*DelH9 - v10(i)*DelH10)*(pellet_flow/(A_furnace_pel*u_s));

        dTdt_g(i) = (m_g(i-1)*Cp_g(i-1))/(rho_g(i)*Cp_g(i)*V_g)*T_g(i-1) - m_g(i)/(rho_g(i)*V_g)*T_g(i)...   
        - ((h_sg(i)*a_b)/(rho_g(i)*Cp_g(i)*eps_bed))*(T_g(i)-T_s(i))...
        - ((U_wall(i)*A_wall)/(rho_g(i)*Cp_g(i)*V_g))*(T_g(i)-T_amb)...
        + (1/(rho_g(i)*Cp_g(i)))*(-v7(i)*DelH7(i) - v8(i)*DelH8(i))*(pellet_flow/(A_furnace_pel*u_s));

    end

end

% Energy balance check, MW
% if all heats of rxns are zero Qbal should be zero except for heat lost to
% environment through U_wall, but this is small

Q_gin = (m_gin*Cp_gin*T_gin)/1e6;
Q_sin = (m_sin*Cp_sin*T_sin)/1e6;

Q_gout = (m_gout*Cp_g(end)*T_g(end))/1e6;
Q_sout = (m_sin*Cp_s(1)*T_s(1))/1e6;

Q_in = Q_gin + Q_sin;
Q_out = Q_gout + Q_sout;

Q_bal = Q_in - Q_out;

end

== matlab function H2_DRI_plant/DRI Shaft Furnace/solid_conc ==
  data: rho_Fe2O3in output; w_Fe2O3 input; w_Fe3O4 input; w_FeO input; w_Fe input; w_C input; w_Gan input; m_solid input; rho_Fe3O4in output; rho_FeOin output; A_furnace parameter; rho_Fein output; rho_Cin output; rho_Ganin output; u_sin output; rho_p parameter; eps_bed parameter; pellet_flow output; r_p parameter
function [rho_Fe2O3in, rho_Fe3O4in, rho_FeOin, rho_Fein, rho_Cin, rho_Ganin, u_sin, pellet_flow] = solid_conc(w_Fe2O3, w_Fe3O4, w_FeO, w_Fe, w_C, w_Gan, m_solid, A_furnace,rho_p, eps_bed, r_p)

%toal mass concentration using ped porosity and density of pellet
rho_bedin = rho_p; %kg/^3 of SOLID

%mass concentrations of each iron species in
rho_Fe2O3in = rho_bedin * w_Fe2O3; %kg/m^3 of pellet
rho_Fe3O4in = rho_bedin * w_Fe3O4; %kg/m^3 of pellet
rho_FeOin = rho_bedin * w_FeO; %kg/m^3 of pellet
rho_Fein = rho_bedin * w_Fe; %kg/m^3 of pellet
rho_Cin = rho_bedin * w_C; %kg/m^3 of pellet
rho_Ganin = rho_bedin * w_Gan; %kg/m^3 of pellet


%vol_flow = m_solid/(rho_bedin*(1-eps_bed)); %m^3 total/s

u_sup = m_solid/(rho_p*A_furnace);%*(1-eps_bed));

            
u_sin = u_sup/(1-eps_bed);

%interstitial velocity of mass flow, m/s
%u_sin = m_solid/rho_bedin/(A_furnace*(1-eps_bed));


%check this!
pellet_flow = (3*m_solid)/(4*pi*r_p^3*rho_bedin); %pellets/s
